simulink model "TriWave"  (R2022b)
settings: Solver=VariableStepAuto  StartTime=0.0  StopTime=10  MaxStep=1e-3  MinStep=1e-4  RelTol=1e-3
libraries: simulink x3
settings Model: Creator=yeyi5  LastModifiedBy=yeyi5

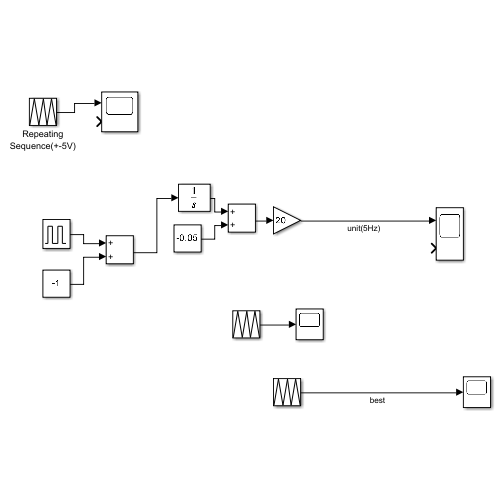
[thumbnail: Simulink's stored preview of the top-level diagram]
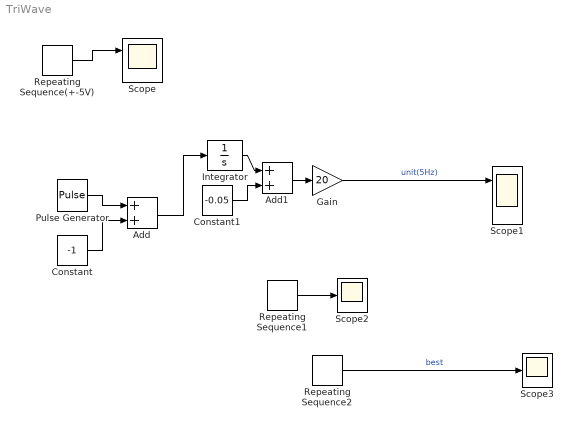
== system TriWave ==
  Add : Sum
  Add1 : Sum
  Constant : Constant  Value=-1
  Constant1 : Constant  Value=-0.05
  Gain : Gain  Gain=20
  Integrator : Integrator
  Pulse Generator : DiscretePulseGenerator  PulseType=Time based  Amplitude=2  Period=1/5  PulseWidth=50
  Repeating Sequence(+-5V) : simulink/Sources/Repeating Sequence  rep_seq_t=[0, 0.1, 0.2]  rep_seq_y=[-5, 5, -5]
  Repeating Sequence1 : simulink/Sources/Repeating Sequence  rep_seq_t=[0, 0.1, 0.2]  rep_seq_y=[-1, 1, -1]
  Repeating Sequence2 : simulink/Sources/Repeating Sequence  rep_seq_t=[0, 0.5/0.5, 1/0.5]  rep_seq_y=[-1, 1, -1]
  Scope : Scope  NumInputPorts=2
  Scope1 : Scope  NumInputPorts=2
  Scope2 : Scope
  Scope3 : Scope
  wires:
  Repeating Sequence(+-5V)/1 -> Scope/1
  Add1/1 -> Gain/1
  Integrator/1 -> Add1/1
  Pulse Generator/1 -> Add/1
  Constant/1 -> Add/2
  Add/1 -> Integrator/1
  Constant1/1 -> Add1/2
  Gain/1 -> Scope1/1  "unit(5Hz)"
  Repeating Sequence1/1 -> Scope2/1
  Repeating Sequence2/1 -> Scope3/1  "best"
